simulink model "no_cntroller_sim"  (R2023a)
settings: Solver=FixedStepAuto  StartTime=0.0  StopTime=Tf  RelTol=1e-3
values from neighbouring files (symbols this model uses):
  vehicle_data = getVehicleDataStruct()    [main.m]
undefined symbols (not defined in the file or in its folder): input
libraries: autolibshared x1
settings Model: Creator=ashkan  LastModifiedBy=ashkan
settings OptimizationCC: ReuseModelBlockBuffer=off

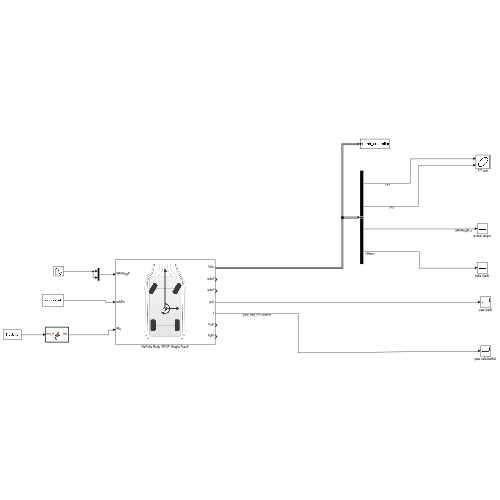
[thumbnail: Simulink's stored preview of the top-level diagram]
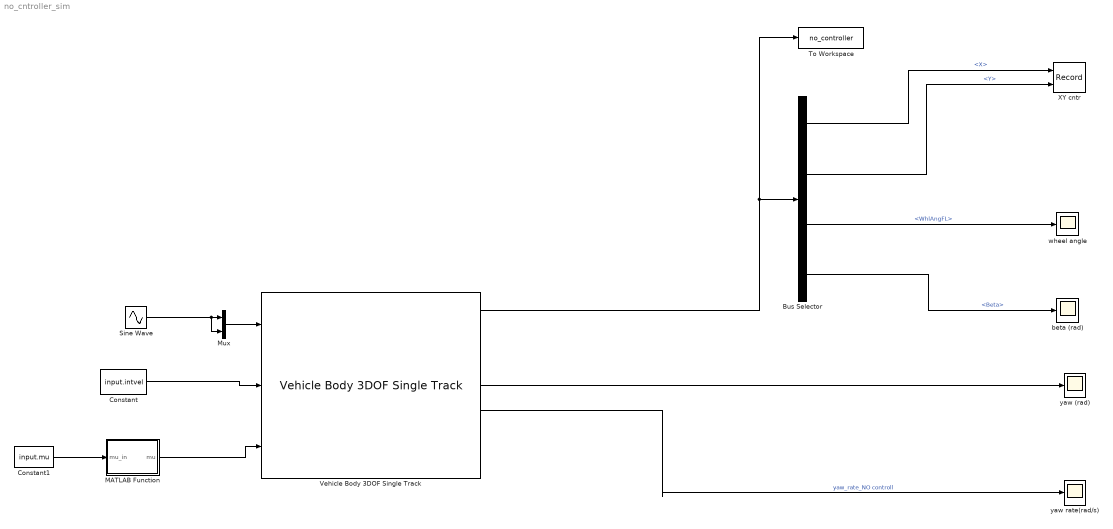
== system no_cntroller_sim ==
  Bus Selector : BusSelector  OutputSignals=InertFrm.Cg.Disp.X,InertFrm.Cg.Disp.Y,BdyFrm.FrntAxl.Steer.WhlAngFL,BdyFrm.Cg.Ang.Beta
  Constant : Constant  Value=input.intvel
  Constant1 : Constant  Value=input.mu
  MATLAB Function : MATLAB Function  TreatAsAtomicUnit=on
  Mux : Mux  Inputs=2
  Sine Wave : Sin  Amplitude=input.str.amp  Frequency=input.str.freq  SampleTime=input.str.sample_time
  To Workspace : ToWorkspace  VariableName=no_controller  SaveFormat=Timeseries  SampleTime=-1
  Vehicle Body 3DOF Single Track : autolibshared/Vehicle Body 3DOF Single Track  trackMode=Dual  inputMode=External longitudinal velocity  frontSteerMode=on  rearSteerMode=off  windMode=off  muMode=on  extFMode=off  extMMode=off  htchFMode=off  htchMMode=off  extXo=off  extpsio=off  extxdoto=off  extro=off  extYo=off  extTamb=off  extydoto=off  aMode=2  NF=2  NR=2  m=vehicle_data.vehicle.m  a=vehicle_data.vehicle.Lf  b=vehicle_data.vehicle.Lr  h=vehicle_data.vehicle.hGs  dh=1  hh=0.2  X_o=0  xdot_o=0  CalphaMode=off  sigmaMode=off  d=0  hl=0  w="[vehicle_data.vehicle.Wf ,  vehicle_data.vehicle.Wr]"  Cy_f=vehicle_data.front_suspension.Ks_f  Cy_r=vehicle_data.rear_suspension.Ks_r  sigma_f=.1  sigma_r=.1  alpha_f_brk=[-.1 .1]  Cy_f_data=[-9e3 9e3]  alpha_r_brk=[-.1 .1]  Cy_r_data=[-9e3 9e3]  Y_o=0  ydot_o=0  Izz=4000  psi_o=0  r_o=0  Af=2  Cd=.3  Cl=.1  Cpm=.1  beta_w=[0 0.01:0.01:0.3]  Cs=[0 0.01:0.01:0.3]  Cym=[0 1e-6:0.01:0.3]  Pabs=101325  Tair=273  g=9.81  mu=1  xdot_tol=.01  Fznom=5000  Fxtire_sat=7e4  Fytire_sat=7e4  longOff=0  latOff=0  vertOff=0  wrapAng=off
  XY cntr : Record  FileSettingsInternal="{\"entries\":[{\"content\":{\"excelSettings\":{\"content\":{},\"type\":\"Streamout.ExcelSettings\"}},\"type\":\"Streamout.FileSettingStorage\",\"uuid\":\"\"}],\"packageUris\":[\"http:\\/\\/schema.mathworks.com\\/mf0\\/streamout_blocks\\/R2020a\"],\"version\":\"1.0\"}"  Layout=[1 1]  SignalsInternal="{\"entries\":[{\"content\":{\"signals\":[{\"content\":{\"blockPath\":[],\"dimensions\":[1],\"domain\":\"\",\"lineColor\":\"#a2142f\",\"plots\":[1],\"port\":1,\"sid\":[\"\"],\"signalID\":27254,\"signalName\":\"<X>\"},\"type\":\"RecordBlkView.Signal\",\"uuid\":\"\"},{\"content\":{\"blockPath\":[],\"dimensions\":[1],\"domain\":\"\",\"lineColor\":\"#139fff\",\"plots\":[1],\"port\":2,\"sid\":[\"\"],\"signalID\":27258,\"signalName\":\"<Y>\"},\"type\":\"RecordBlkView.Signal\",\"uuid\":\"\"}]},\"type\":\"RecordBlkView.InputSignals\",\"uuid\":\"\"}],\"packageUris\":[\"http:\\/\\/schema.mathworks.com\\/mf0\\/streamout_blocks\\/R2020a\"],\"version\":\"1.0\"}"  VisualizationBindings="{\"xyplotplugin\":{\"info\":[{\"series\":[{\"bindingParametersList\":[{\"parameter\":\"X-Axis\",\"signalID\":27254,\"signalName\":\"<X>\"},{\"parameter\":\"Y-Axis\",\"signalID\":27258,\"signalName\":\"<Y>\"}],\"seriesID\":35332}],\"subplotID\":1}]}}"  CompatibilityTag=XY
  beta (rad) : Scope
  wheel angle : Scope
  yaw (rad) : Scope
  yaw rate(rad/s) : Scope
  wires:
  Bus Selector/2 -> XY cntr/2  "<Y>"
  Bus Selector/3 -> wheel angle/1  "<WhlAngFL>"
  Bus Selector/1 -> XY cntr/1  "<X>"
  Bus Selector/4 -> beta (rad)/1  "<Beta>"
  Vehicle Body 3DOF Single Track/5 -> yaw rate(rad/s)/1  "yaw_rate_NO controll"
  Vehicle Body 3DOF Single Track/1 -> Bus Selector/1, To Workspace/1
  Vehicle Body 3DOF Single Track/4 -> yaw (rad)/1
  Constant/1 -> Vehicle Body 3DOF Single Track/2
  Sine Wave/1 -> Mux/2, Mux/1
  Mux/1 -> Vehicle Body 3DOF Single Track/1
  MATLAB Function/1(mu) -> Vehicle Body 3DOF Single Track/3
  Constant1/1 -> MATLAB Function/1(mu_in)

== matlab function no_cntroller_sim/MATLAB Function ==
  data: mu_in input; mu output
function mu = fcn(mu_in)

mu = mu_in*ones(2);
